simulink model "Teste_potenciometros"  (R2018a)
settings: Solver=FixedStepAuto  StartTime=0.0  StopTime=70  FixedStep=0.0025  RelTol=1e-3  EnableMultiTasking=on
values from neighbouring files (symbols this model uses):
  Pphi = polyfit(phi,y_phi,2)    [Pot.m]
  Pteta = polyfit(teta,y_teta,2)    [Pot.m]
undefined symbols (not defined in the file or in its folder): sigbuilder_block
libraries: arduinolib x4, simulink x1
settings Model: SimulationMode=external  ExtModeTrigDuration=2  Creator=stayn  LastModifiedBy=stayn
settings OptimizationCC: EnhancedBackFolding=on  PassReuseOutputArgsAs=Individual arguments  MaxStackSize=64  OptimizeBlockOrder=speed  DifferentSizesBufferReuse=on  OptimizationCustomize=off
settings DebuggingCC: ParameterTunabilityLossMsg=error
settings HardwareCC: ProdBitPerInt=16  ProdBitPerPointer=16  ProdBitPerSizeT=16  ProdBitPerPtrDiffT=16  ProdLargestAtomicFloat=None  ProdWordSize=8  ProdHWDeviceType=Atmel->AVR
settings SFSimCC: MATLABDynamicMemAlloc=off
settings RTWCC: SystemTargetFile=ert.tlc  HardwareBoard=Arduino Mega 2560  TLCOptions=-aInlineSetEventsForThisBaseRateFcn=TLC_FALSE -aSuppressMultiTaskScheduler=TLC_FALSE -aRateBasedStepFcn=1  TemplateMakefile=ert_default_tmf  GenerateReport=on  Toolchain=Arduino AVR  BuildConfiguration=Faster Runs  IncludeHyperlinkInReport=on  LaunchReport=on  GenerateTraceInfo=on  GenerateTraceReport=on  GenerateTraceReportSl=on  GenerateTraceReportSf=on  GenerateTraceReportEml=on
settings CodeAppCC: ForceParamTrailComments=on  IgnoreCustomStorageClasses=off  OperatorAnnotations=on  SimulinkDataObjDesc=on  SFDataObjDesc=on  InsertBlockDesc=on
settings ERTTargetCC: SupportContinuousTime=on  SupportVariableSizeSignals=on

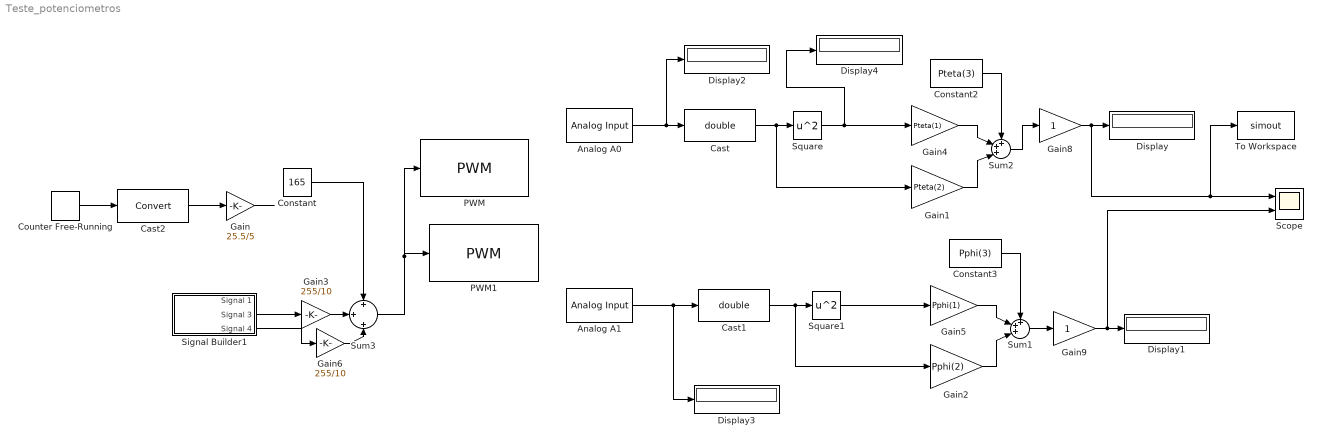
== system Teste_potenciometros ==
  Analog A0 : arduinolib/Analog Input  pinNumber=0  ReadResultsOnly=off  ConversionTriggerSource=Software  ExternalTriggerType=uint32(0)  OutputDataType=uint16  EnableConversionCompleteNotify=off  EnableOuputStatus=off  SampleTime=0.025  blockPlatform=arduino
  Analog A1 : arduinolib/Analog Input  pinNumber=1  ReadResultsOnly=off  ConversionTriggerSource=Software  ExternalTriggerType=uint32(0)  OutputDataType=uint16  EnableConversionCompleteNotify=off  EnableOuputStatus=off  SampleTime=-1  blockPlatform=arduino
  Cast : DataTypeConversion  OutDataTypeStr=double
  Cast1 : DataTypeConversion  OutDataTypeStr=double
  Cast2 : DataTypeConversion
  Constant : Constant  Value=165
  Constant2 : Constant  Value=Pteta(3)
  Constant3 : Constant  Value=Pphi(3)
  Counter Free-Running : simulink/Sources/Counter Free-Running  NumBits=10  tsamp=5
  Display{,1..4} (5 alike) : Display
  Gain : Gain  Gain=25.5/5
  Gain1 : Gain  Gain=Pteta(2)
  Gain2 : Gain  Gain=Pphi(2)
  Gain3 : Gain  Gain=255/10
  Gain4 : Gain  Gain=Pteta(1)
  Gain5 : Gain  Gain=Pphi(1)
  Gain6 : Gain  Gain=255/10
  Gain8 : Gain
  Gain9 : Gain
  PWM : arduinolib/PWM  pinNumber=9  EnableInputFrequency=off  InitialFrequency=2000  InitialDutyCycle=0  NotificationType=None  blockPlatform=arduino
  PWM1 : arduinolib/PWM  pinNumber=8  EnableInputFrequency=off  InitialFrequency=2000  InitialDutyCycle=0  NotificationType=None  blockPlatform=arduino
  Scope : Scope  NumInputPorts=2
  Signal Builder1 : Subsystem  Tag=STV Subsys  LoadFcn=sigbuilder_block('load');  StartFcn=sigbuilder_block('start');  StopFcn=sigbuilder_block('stop');  ClipboardFcn=sigbuilder_block('clipboard');  mask(Sigbuilder block){tuvar=[0:10]}
      mask help: Simulink:masks:SigbuilderBlock_MD
      mask init:
      | if ~strcmp(get_param(bdroot(gcbh),'SimulationStatus'),'stopped') tuvar = sigbuilder_block('maskInit'); end
      settings: CopyFcn=sigbuilder_block('copy');  DeleteFcn=sigbuilder_block('delete');  ModelCloseFcn=sigbuilder_block('modelClose');  PreSaveFcn=sigbuilder_block('preSave');  PauseFcn=sigbuilder_block('pause');  ContinueFcn=sigbuilder_block('continue');  NameChangeFcn=sigbuilder_block('namechange');  OpenFcn=sigbuilder_block('open',[6 30 1012.5 447.75 ]);  CloseFcn=sigbuilder_block('close');
      mask Display: plot(0, 0, 100, 100,[2, 2, 32, 32, 2], [68, 8, 8, 68, 68],[32, 2], [38, 38], [32, 19, 2],[53, 60, 44], [32, 17, 17, 2],[16, 16, 31, 31]);txt = getActiveGroup(gcbh);text(2, 100, txt,'verticalAlignment', 'top');
  Square : Math  Operator=square  SaturateOnIntegerOverflow=on
  Square1 : Math  Operator=square  SaturateOnIntegerOverflow=on
  Sum1 : Sum  Inputs=+++|
  Sum2 : Sum  Inputs=+++|
  Sum3 : Sum  Inputs=+|+|+
  To Workspace : ToWorkspace  VariableName=simout  SampleTime=-1
      settings: Save2DSignal=2-D array (concatenate along first dimension)
  wires:
  Gain8/1 -> To Workspace/1, Scope/1, Display/1
  Gain9/1 -> Scope/2, Display1/1
  Gain4/1 -> Sum2/2
  Analog A0/1 -> Cast/1, Display2/1
  Constant2/1 -> Sum2/1
  Sum2/1 -> Gain8/1
  Analog A1/1 -> Display3/1, Cast1/1
  Cast/1 -> Gain1/1, Square/1
  Gain1/1 -> Sum2/3
  Square/1 -> Display4/1, Gain4/1
  Gain2/1 -> Sum1/3
  Constant3/1 -> Sum1/1
  Cast1/1 -> Gain2/1, Square1/1
  Gain5/1 -> Sum1/2
  Square1/1 -> Gain5/1
  Sum1/1 -> Gain9/1
  Cast2/1 -> Gain/1
  Gain/1 -> ?
  Counter Free-Running/1 -> Cast2/1
  Sum3/1 -> PWM/1, PWM1/1
  Signal Builder1/2(Signal 3) -> Gain3/1
  Signal Builder1/3(Signal 4) -> Gain6/1
  Constant/1 -> Sum3/1
  Gain3/1 -> Sum3/2
  Gain6/1 -> Sum3/3

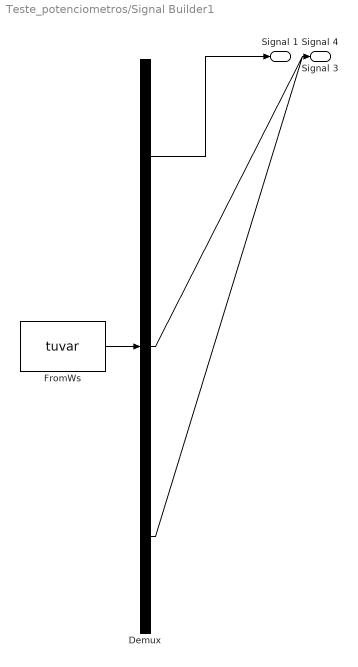
== system Teste_potenciometros/Signal Builder1 ==
  Demux : Demux  Tag=STV Demux  Outputs=3
  FromWs : FromWorkspace  Tag=STV FromWs  VariableName=tuvar  SampleTime=0
      SigBuilderData=|
      | common.afterFinalStr = 'Extrapolate'
      | common.sampleTime = 0
      | dataSet.timeRange = [0 100]
      | dataSet.name = 'Group 1'
      | sbobj.Groups.Name = 'Group 1'
      | sbobj.Groups.Signals(1).Name = 'Signal 1'
      | sbobj.Groups.Signals(1).XData = [0 0.0005 0.0005 90 90 100]
      | sbobj.Groups.Signals(1).YData = [0 0 2.5 2.5 0 0]
      | sbobj.Groups.Signals(2).Name = 'Signal 3'
      | sbobj.Groups.Signals(2).XData = [0 15.1 15.1 30 30 100]
      | sbobj.Groups.Signals(2).YData = [0 0 0.5 0.5 0 0]
      | sbobj.Groups.Signals(3).Name = 'Signal 4'
      | sbobj.Groups.Signals(3).XData = [0 45 45 60 60 100]
      | sbobj.Groups.Signals(3).YData = [0 0 -0.5 -0.5 0 0]
      | sbobj.Groups.TimeRange = [0 100]
  Signal 1 : Outport  Tag=STV Outport
  Signal 3 : Outport  Tag=STV Outport  Port=2
  Signal 4 : Outport  Tag=STV Outport  Port=3
  wires:
  Demux/1 -> Signal 1/1
  FromWs/1 -> Demux/1
  Demux/2 -> Signal 3/1
  Demux/3 -> Signal 4/1
